simulink model "ASSIG2_v1"  (R2020a)
settings: Solver=FixedStepAuto  StartTime=0.0  StopTime=10.0  FixedStep=1e-3  RelTol=1e-3  EnableMultiTasking=on
undefined symbols (not defined in the file): D0, D1, D10, D11, D12, D13, D2, D3, D4, D5, D6, D7, D8, D9, PTA0, PTA1, PTA2, PTB23, PTB9, PTC16, PTC17, PTC2, PTC3, PTC4, PTD0, PTD1, PTD2, PTD3
libraries: frdmk64flib x14
settings Model: ExtModeTrigDuration=5  Creator=Nour  LastModifiedBy=Khaled
settings OptimizationCC: EnhancedBackFolding=on  PassReuseOutputArgsAs=Individual arguments  ZeroExternalMemoryAtStartup=off  ZeroInternalMemoryAtStartup=off  MaxStackSize=64  OptimizeBlockOrder=speed  DifferentSizesBufferReuse=on  OptimizationCustomize=off  EfficientTunableParamExpr=on
settings DebuggingCC: ParameterTunabilityLossMsg=error
settings HardwareCC: ProdBitPerPointer=32  ProdBitPerSizeT=32  ProdBitPerPtrDiffT=32  ProdLargestAtomicInteger=Long  ProdLargestAtomicFloat=Double  ProdWordSize=32  ProdHWDeviceType=ARM Compatible->ARM Cortex
settings SFSimCC: MATLABDynamicMemAlloc=off
settings RTWCC: SystemTargetFile=ert.tlc  HardwareBoard=NXP FRDM-K64F  TemplateMakefile=ert_default_tmf  Toolchain=GNU Tools for ARM Embedded Processors
settings CodeAppCC: ForceParamTrailComments=on  IgnoreCustomStorageClasses=off  OperatorAnnotations=on  SimulinkDataObjDesc=on  SFDataObjDesc=on  InsertBlockDesc=on

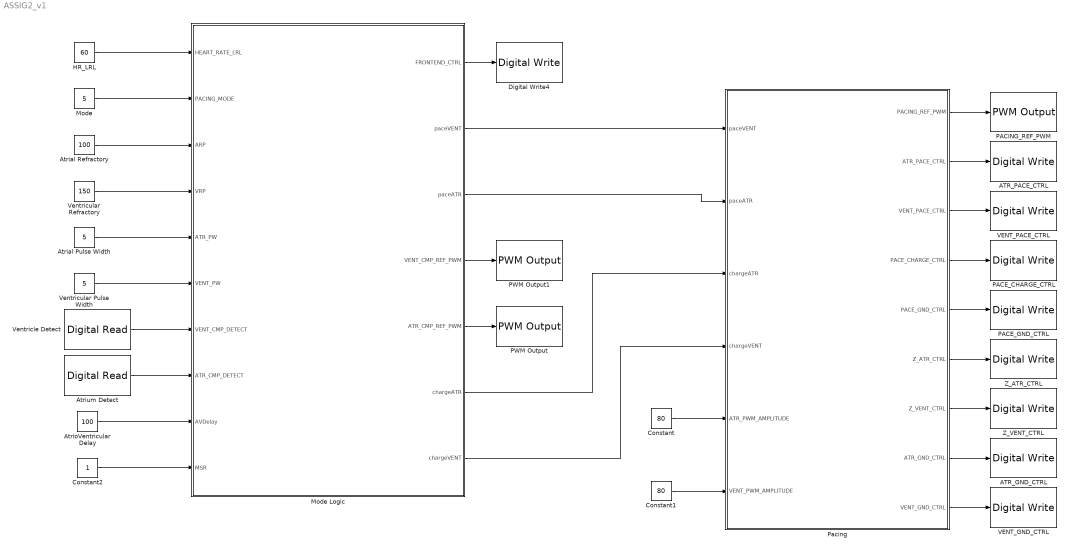
== system ASSIG2_v1 ==
  ATR_GND_CTRL : frdmk64flib/Digital Write  Whichpin=PTD2 (D11)
  ATR_PACE_CTRL : frdmk64flib/Digital Write  Whichpin=PTA0 (D8)
  Atrial Pulse Width : Constant  Value=5  OutDataTypeStr=uint16
  Atrial Refractory : Constant  Value=100  OutDataTypeStr=uint16
  AtrioVentricular Delay : Constant  Value=100  OutDataTypeStr=uint16
  Atrium Detect : frdmk64flib/Digital Read  Whichpin=PTC16 (D0)  SampleTime=-1
  Constant : Constant  Value=80  OutDataTypeStr=uint16
  Constant1 : Constant  Value=80  OutDataTypeStr=uint16
  Constant2 : Constant  OutDataTypeStr=uint16
  Digital Write4 : frdmk64flib/Digital Write  Whichpin=PTD1 (D13)
  HR_LRL : Constant  Value=60  OutDataTypeStr=uint16
  Mode : Constant  Value=5  OutDataTypeStr=uint16
  Mode Logic : Stateflow chart  TreatAsAtomicUnit=on
  PACE_CHARGE_CTRL : frdmk64flib/Digital Write  Whichpin=PTB9 (D2)
  PACE_GND_CTRL : frdmk64flib/Digital Write  Whichpin=PTD0 (D10)
  PACING_REF_PWM : frdmk64flib/PWM Output  Whichpin=PTA2 (D5)  InitialFrequency=2000  InitialDutyCycle=80
  PWM Output : frdmk64flib/PWM Output  Whichpin=PTC2 (D6)  InitialFrequency=2000  InitialDutyCycle=20
  PWM Output1 : frdmk64flib/PWM Output  Whichpin=PTA1 (D3)  InitialFrequency=2000  InitialDutyCycle=20
  Pacing : Stateflow chart  TreatAsAtomicUnit=on
  VENT_GND_CTRL : frdmk64flib/Digital Write  Whichpin=PTD3 (D12)
  VENT_PACE_CTRL : frdmk64flib/Digital Write  Whichpin=PTC4 (D9)
  Ventricle Detect : frdmk64flib/Digital Read  Whichpin=PTC17 (D1)  SampleTime=-1
  Ventricular Pulse Width : Constant  Value=5  OutDataTypeStr=uint16
  Ventricular Refractory : Constant  Value=150  OutDataTypeStr=uint16
  Z_ATR_CTRL : frdmk64flib/Digital Write  Whichpin=PTB23 (D4)
  Z_VENT_CTRL : frdmk64flib/Digital Write  Whichpin=PTC3 (D7)
  wires:
  Pacing/1(PACING_REF_PWM) -> PACING_REF_PWM/1
  Pacing/2(ATR_PACE_CTRL) -> ATR_PACE_CTRL/1
  Pacing/3(VENT_PACE_CTRL) -> VENT_PACE_CTRL/1
  Pacing/4(PACE_CHARGE_CTRL) -> PACE_CHARGE_CTRL/1
  Pacing/5(PACE_GND_CTRL) -> PACE_GND_CTRL/1
  Pacing/6(Z_ATR_CTRL) -> Z_ATR_CTRL/1
  Pacing/7(Z_VENT_CTRL) -> Z_VENT_CTRL/1
  Pacing/8(ATR_GND_CTRL) -> ATR_GND_CTRL/1
  Pacing/9(VENT_GND_CTRL) -> VENT_GND_CTRL/1
  Mode Logic/1(FRONTEND_CTRL) -> Digital Write4/1
  Mode Logic/2(paceVENT) -> Pacing/1(paceVENT)
  Mode Logic/3(paceATR) -> Pacing/2(paceATR)
  HR_LRL/1 -> Mode Logic/1(HEART_RATE_LRL)
  Mode/1 -> Mode Logic/2(PACING_MODE)
  Atrial Refractory/1 -> Mode Logic/3(ARP)
  Ventricular Refractory/1 -> Mode Logic/4(VRP)
  Atrial Pulse Width/1 -> Mode Logic/5(ATR_PW)
  Ventricle Detect/1 -> Mode Logic/7(VENT_CMP_DETECT)
  Atrium Detect/1 -> Mode Logic/8(ATR_CMP_DETECT)
  Mode Logic/4(VENT_CMP_REF_PWM) -> PWM Output1/1
  Mode Logic/5(ATR_CMP_REF_PWM) -> PWM Output/1
  Ventricular Pulse Width/1 -> Mode Logic/6(VENT_PW)
  Mode Logic/6(chargeATR) -> Pacing/3(chargeATR)
  Mode Logic/7(chargeVENT) -> Pacing/4(chargeVENT)
  Constant/1 -> Pacing/5(ATR_PWM_AMPLITUDE)
  Constant1/1 -> Pacing/6(VENT_PWM_AMPLITUDE)
  AtrioVentricular Delay/1 -> Mode Logic/9(AVDelay)
  Constant2/1 -> Mode Logic/10(MSR)

== stateflow chart ASSIG2_v1/Mode Logic ==
  state AAI
    state Charge
      entry:
      paceATR = false;
      paceVENT = false;
      chargeVENT = false;
      chargeATR = true;
      FRONTEND_CTRL = true;
    state Pace
      entry:
      chargeATR = false;
      chargeVENT = false;
      paceVENT = false;
      paceATR = true;
      FRONTEND_CTRL = true;
    state Refractor
      entry:
      paceATR = false;
      paceVENT = false;
      chargeVENT = false;
      chargeATR = true;
      FRONTEND_CTRL = true;
    (default) -> AAI.Charge
    AAI.Charge -> AAI.Pace [order 1] : [after((60000 / HEART_RATE_LRL - ARP - delay), msec)]
    AAI.Charge -> AAI.Refractor [order 2] : [ATR_CMP_DETECT == true]{delay = 0}
    AAI.Refractor -> AAI.Charge : [after(ARP, msec)]
    AAI.Pace -> AAI.Refractor : [after(ATR_PW, msec)]{delay = ATR_PW}
  state Entry
    %% PACING_MODE Values:
    %% 1: AOO
    %% 2: VOO
    %% 3: AAI
    %% 4: VVI
    %% 5: DOO
    entry:
    ATR_CMP_REF_PWM = 80;
    VENT_CMP_REF_PWM = 20;
    delay = 0;
  state AOO
    state PACE
      entry:
      chargeATR = false;
      chargeVENT = false;
      paceVENT = false;
      paceATR = true;
    state CHARGE
      entry:
      paceATR = false;
      paceVENT = false;
      chargeVENT = false;
      chargeATR = true;
    AOO.PACE -> AOO.CHARGE : [after(ATR_PW, msec)]
    (default) -> AOO.PACE
    AOO.CHARGE -> AOO.PACE : [after((60000 / HEART_RATE_LRL - ATR_PW), msec)]
  state VVI
    state Charge
      entry:
      paceATR = false;
      paceVENT = false;
      chargeATR = false;
      chargeVENT = true;
      FRONTEND_CTRL = true;
    state Pace
      entry:
      chargeATR = false;
      chargeVENT = false;
      paceATR = false;
      paceVENT = true;
      FRONTEND_CTRL = true;
    state Refractor
      entry:
      paceATR = false;
      paceVENT = false;
      chargeATR = false;
      chargeVENT = true;
      FRONTEND_CTRL = true;
    (default) -> VVI.Charge
    VVI.Charge -> VVI.Pace [order 1] : [after((60000 / HEART_RATE_LRL - VRP - delay), msec)]
    VVI.Charge -> VVI.Refractor [order 2] : [VENT_CMP_DETECT == true]{delay = 0}
    VVI.Refractor -> VVI.Charge : [after(VRP, msec)]
    VVI.Pace -> VVI.Refractor : [after(VENT_PW, msec)]{delay = VENT_PW}
  state VOO
    state PACE
      entry:
      chargeATR = false;
      chargeVENT = false;
      paceATR = false;
      paceVENT = true;
    state CHARGE
      entry:
      paceATR = false;
      paceVENT = false;
      chargeATR = false;
      chargeVENT = true;
    VOO.PACE -> VOO.CHARGE : [after(ATR_PW, msec)]
    (default) -> VOO.PACE
    VOO.CHARGE -> VOO.PACE : [after((60000 / HEART_RATE_LRL - ATR_PW), msec)]
  state DOO
    state ATRCharge
      entry:
      paceATR = false;
      paceVENT = false;
      chargeATR = true;
      chargeVENT = false;
    state ATRPace
      entry:
      paceATR = true;
      paceVENT = false;
      chargeATR = false;
      chargeVENT = false;
    state VentPace
      entry:
      paceATR = false;
      paceVENT = true;
      chargeATR = false;
      chargeVENT = false;
    state VENTCharge
      entry:
      paceATR = false;
      paceVENT = false;
      chargeATR = false;
      chargeVENT = true;
    (default) -> ATRCharge
    ATRCharge -> ATRPace : [after((60000 / HEART_RATE_LRL - AVDelay - ATR_PW - VENT_PW), msec)]
    ATRPace -> VENTCharge : [after(ATR_PW, msec)]
    VentPace -> ATRCharge : [after(VENT_PW, msec)]
    VENTCharge -> VentPace : [after(AVDelay, msec)]
  (default) -> Entry
  Entry -> AAI [order 3] : [PACING_MODE == 3]
  Entry -> AOO [order 1] : [PACING_MODE == 1]
  AAI -> Entry : [PACING_MODE ~= 3]
  AOO -> Entry : [PACING_MODE ~= 1]
  Entry -> VVI [order 4] : [PACING_MODE == 4]
  Entry -> VOO [order 2] : [PACING_MODE == 2]
  VVI -> Entry : [PACING_MODE ~= 4]
  VOO -> Entry : [PACING_MODE ~= 2]
  Entry -> DOO [order 5] : [PACING_MODE == 5]
  DOO -> Entry : [PACING_MODE ~= 5]
  data: FRONTEND_CTRL output boolean; paceVENT output boolean; paceATR output boolean; delay local uint16; HEART_RATE_LRL input uint16; PACING_MODE input uint16; VENT_CMP_REF_PWM output uint16; ATR_CMP_REF_PWM output uint16; ARP input uint16; VRP input uint16; ATR_PW input uint16; VENT_PW input uint16; VENT_CMP_DETECT input boolean; ATR_CMP_DETECT input boolean; chargeATR output boolean; chargeVENT output boolean; AVDelay input uint16; MSR input uint16

== stateflow chart ASSIG2_v1/Pacing ==
  state ENTRY_STATE
    %% Reset all values
    %% to 0 or false
    entry:
    ATR_PACE_CTRL = false;
    VENT_PACE_CTRL = false;
    PACING_REF_PWM = 0;
    PACE_CHARGE_CTRL = false;
    PACE_GND_CTRL = false;
    Z_ATR_CTRL = false;
    Z_VENT_CTRL = false;
    ATR_GND_CTRL = false;
    VENT_GND_CTRL = false;
  state CHARGE_VENT2PACE_VENT
    %% Charge C22, Discharge C21
    entry:
    ATR_PACE_CTRL = false;
    VENT_PACE_CTRL = false;
    PACING_REF_PWM = VENT_PWM_AMPLITUDE;
    PACE_CHARGE_CTRL = true;
    %Dishcharging Blocking Capacitor
    PACE_GND_CTRL = true;
    Z_ATR_CTRL = false;
    Z_VENT_CTRL = false;
    ATR_GND_CTRL = false;
    VENT_GND_CTRL = true;
  state Charge_Atr_Paced_Atr
    %Charge C22 for atrial pulse
    %Just recieved atrial pulse
    entry:
    ATR_PACE_CTRL = false;
    VENT_PACE_CTRL = false;
    PACING_REF_PWM = ATR_PWM_AMPLITUDE;
    PACE_CHARGE_CTRL = true;
    %Discharging Blocking Capacitor
    PACE_GND_CTRL = true;
    Z_ATR_CTRL = false;
    Z_VENT_CTRL = false;
    ATR_GND_CTRL = true;
    VENT_GND_CTRL = false;
  state pace_ventricle
    entry:
    %% Pacing the ventricle
    PACE_CHARGE_CTRL = false;
    PACE_GND_CTRL = true;
    ATR_PACE_CTRL = false;
    ATR_GND_CTRL = false;
    Z_ATR_CTRL = false;
    Z_VENT_CTRL = false;
    VENT_GND_CTRL = false;
    VENT_PACE_CTRL = true;
  state pace_atrium
    entry:
    %% Pacing the atrium
    PACE_CHARGE_CTRL = false;
    PACE_GND_CTRL = true;
    ATR_PACE_CTRL = true;
    ATR_GND_CTRL = false;
    Z_ATR_CTRL = false;
    Z_VENT_CTRL = false;
    VENT_GND_CTRL = false;
    VENT_PACE_CTRL = false;
  (default) -> ENTRY_STATE
  ENTRY_STATE -> CHARGE_VENT2PACE_VENT [order 1] : [chargeVENT == true]
  ENTRY_STATE -> Charge_Atr_Paced_Atr [order 2] : [chargeATR == true]
  pace_atrium -> ENTRY_STATE [order 2] : [chargeATR == false]
  pace_ventricle -> ENTRY_STATE [order 2] : [chargeVENT == false]
  CHARGE_VENT2PACE_VENT -> pace_ventricle : [paceVENT == true]
  pace_ventricle -> CHARGE_VENT2PACE_VENT [order 1] : [chargeVENT == true]
  pace_atrium -> Charge_Atr_Paced_Atr [order 1] : [chargeATR == true]
  Charge_Atr_Paced_Atr -> pace_atrium : [paceATR == true]
  data: PACING_REF_PWM output uint16; ATR_PACE_CTRL output boolean; VENT_PACE_CTRL output boolean; PACE_CHARGE_CTRL output boolean; PACE_GND_CTRL output boolean; Z_ATR_CTRL output boolean; Z_VENT_CTRL output boolean; ATR_GND_CTRL output boolean; VENT_GND_CTRL output boolean; paceVENT input boolean; paceATR input boolean; chargeATR input boolean; chargeVENT input boolean; ATR_PWM_AMPLITUDE input uint16; VENT_PWM_AMPLITUDE input uint16
